simulink model "PEMFC_system"  (R2014b)
settings: Solver=ode45  StartTime=0.0  StopTime=10.0  RelTol=1e-3
settings Model: Creator=DELL  LastModifiedBy=dell

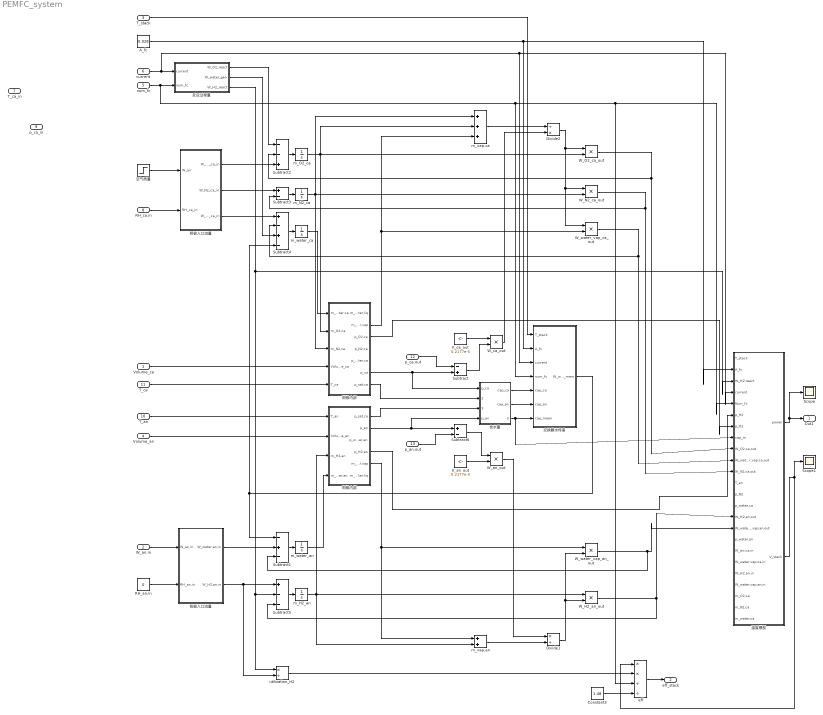
== system PEMFC_system ==
  Volume_ca : Inport
  W_an,in : Inport  Port=2
  T_stack : Inport  Port=3
  Volume_an : Inport  Port=4
  num_fc : Inport  Port=5
  current : Inport  Port=6
  T_ca_in : Inport  Port=7
  RH_ca,in : Inport  Port=8
  p_ca_in : Inport  Port=9
  T_an : Inport  Port=10
  T_ca : Inport  Port=11
  p_ca,out : Inport  Port=12
  p_an,out : Inport  Port=13
  A_fc : Constant  Value=0.028
  Constant3 : Constant  Value=1.48
  Divide1 : Product  Inputs=*/
  Divide2 : Product  Inputs=/*
  K_an_out : Constant  Value=0.2177e-5
  K_ca_out : Constant  Value=0.2177e-5
  RH_an,in : Constant  Value=0
  Scope : Scope
  Scope1 : Scope
  Subtract : Sum  Inputs=-+
  Subtract1 : Sum  Inputs=-+-
  Subtract2 : Sum  Inputs=--+
  Subtract3 : Sum  Inputs=+-
  Subtract4 : Sum  Inputs=+-+-
  Subtract5 : Sum  Inputs=+--
  Subtract6 : Sum  Inputs=+-
  W_H2_an_out : Product
  W_N2_ca_out : Product
  W_O2_ca_out : Product
  W_an_out : Product
  W_ca_out : Product
  W_water_vap_an_out : Product
  W_water_vap_ca_out : Product
  eff : Product  Inputs=**//
  m_H2_an : Integrator
  m_N2_ca : Integrator
  m_O2_ca : Integrator
  m_vap,an : Sum
  m_vap,ca : Sum  Inputs=+++
  m_water_an : Integrator
  m_water_ca : Integrator
  utilization_H2 : Product  Inputs=*/
  交换膜水传递 : Subsystem  TreatAsAtomicUnit=on
  反应过程量 : Subsystem
  含水量 : Subsystem
  温度模型 : Subsystem
  空气质量 : Step  SampleTime=0
  阳极入口流量 : Subsystem
  阳极内部 : Subsystem
  阴极入口流量 : Subsystem  TreatAsAtomicUnit=on
  阴极内部 : Subsystem
  Out1 : Outport
  eff_stack : Outport  Port=2
  wires:
  温度模型/1(power) -> Scope/1, Out1/1
  温度模型/2(V_stack) -> Scope1/1, eff/1
  current/1 -> 温度模型/4(current), 交换膜水传递/3(current), 反应过程量/1(current)
  Volume_ca/1 -> 阴极内部/4(Volume_ca)
  阴极内部/6(p_ca) -> 含水量/1(p_ca), Subtract/2
  Subtract/1 -> W_ca_out/2
  K_ca_out/1 -> W_ca_out/1
  阴极入口流量/1(W_O2_ca_in) -> Subtract2/3
  反应过程量/3(W_H2_react) -> utilization_H2/1, Subtract5/2, 温度模型/3(W_H2,react)
  反应过程量/1(W_O2_react) -> Subtract2/1
  Subtract2/1 -> m_O2_ca/1
  阴极入口流量/2(W_N2_ca_in) -> Subtract3/1
  Subtract3/1 -> m_N2_ca/1
  阴极入口流量/3(W_water_ca_in) -> Subtract4/1
  Subtract4/1 -> m_water_ca/1
  反应过程量/2(W_water_gen) -> Subtract4/3
  m_O2_ca/1 -> W_O2_ca_out/2, m_vap,ca/2, 阴极内部/2(m_O2,ca)
  m_N2_ca/1 -> W_N2_ca_out/2, m_vap,ca/1, 阴极内部/3(m_N2,ca)
  T_stack/1 -> 交换膜水传递/1(T_stack)
  阴极内部/2(m_water,vap) -> W_water_vap_ca_out/2, m_vap,ca/3
  m_water_ca/1 -> 阴极内部/1(m_water,ca)
  m_vap,ca/1 -> Divide2/1
  W_ca_out/1 -> Divide2/2
  Divide2/1 -> W_water_vap_ca_out/1, W_N2_ca_out/1, W_O2_ca_out/1
  W_O2_ca_out/1 -> 温度模型/9(W_O2,ca,out), Subtract2/2
  W_N2_ca_out/1 -> 温度模型/11(W_N2,ca,out), Subtract3/2
  W_water_vap_ca_out/1 -> Subtract4/2, 温度模型/10(W_water,vap,ca,out)
  交换膜水传递/1(W_water_mem) -> Subtract1/1, Subtract4/4
  W_an,in/1 -> 阳极入口流量/1(W_an,in)
  RH_an,in/1 -> 阳极入口流量/2(RH_an,in)
  阳极入口流量/2(W_H2,an,in) -> utilization_H2/2, Subtract5/1
  Subtract5/1 -> m_H2_an/1
  Subtract1/1 -> m_water_an/1
  阳极内部/4(p_H2,an) -> 温度模型/6(p_H2)
  Volume_an/1 -> 阳极内部/2(Volume_an)
  Subtract6/1 -> W_an_out/1
  K_an_out/1 -> W_an_out/2
  阳极内部/5(m_water,vap) -> W_water_vap_an_out/1, m_vap,an/1
  m_H2_an/1 -> W_H2_an_out/1, m_vap,an/2, 阳极内部/3(m_H2,an)
  W_an_out/1 -> Divide1/1
  m_vap,an/1 -> Divide1/2
  m_water_an/1 -> 阳极内部/4(m_water,an)
  Divide1/1 -> W_water_vap_an_out/2, W_H2_an_out/2
  阳极入口流量/1(W_water,an,in) -> Subtract1/2
  W_water_vap_an_out/1 -> 温度模型/16(W_water,vap,an,out), Subtract1/3
  W_H2_an_out/1 -> Subtract5/3, 温度模型/15(W_H2,an,out)
  阳极内部/2(p_an) -> Subtract6/1, 含水量/4(p_an)
  含水量/3(cap_mean) -> 交换膜水传递/7(cap_mean), 温度模型/8(cap_m)
  含水量/1(cap_ca) -> 交换膜水传递/5(cap_ca)
  含水量/2(cap_an) -> 交换膜水传递/6(cap_an)
  A_fc/1 -> 温度模型/2(A_fc), 交换膜水传递/2(A_fc)
  utilization_H2/1 -> eff/2
  num_fc/1 -> 反应过程量/2(num_fc), 交换膜水传递/4(num_fc), 温度模型/5(Num_fc), eff/3
  Constant3/1 -> eff/4
  eff/1 -> eff_stack/1
  空气质量/1 -> 阴极入口流量/1(W_air)
  阴极内部/3(p_O2,ca) -> 温度模型/7(p_O2)
  RH_ca,in/1 -> 阴极入口流量/2(RH_ca_in)
  T_an/1 -> 阳极内部/1(T_an)
  T_ca/1 -> 阴极内部/5(T_ca)
  阴极内部/7(p_sat,ca) -> 含水量/2(p_sat,ca)
  阳极内部/1(p_sat,ca) -> 含水量/3(p_sat,an)
  p_ca,out/1 -> Subtract/1
  p_an,out/1 -> Subtract6/2

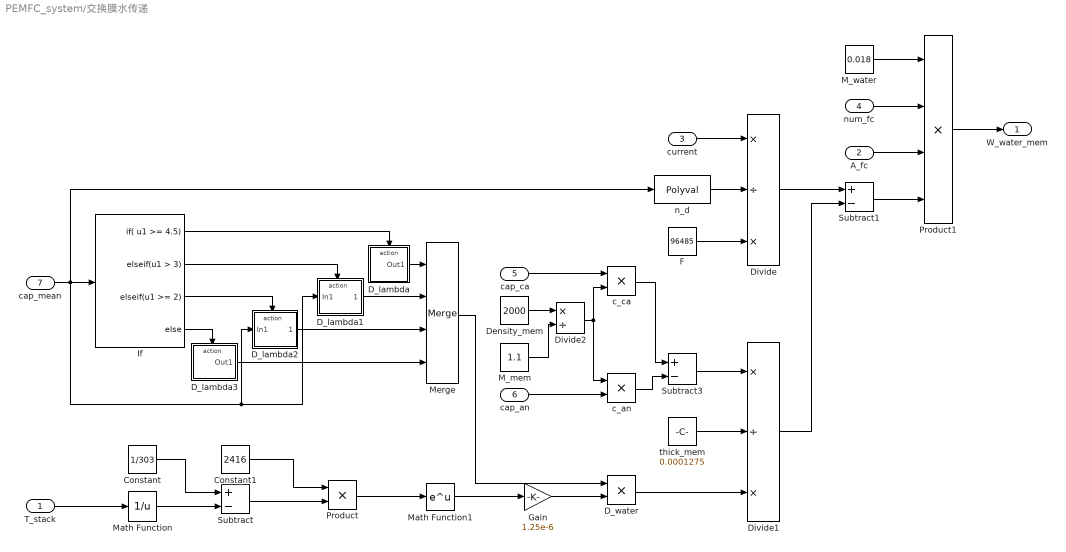
== system PEMFC_system/交换膜水传递 ==
  T_stack : Inport
  A_fc : Inport  Port=2
  current : Inport  Port=3
  num_fc : Inport  Port=4
  cap_ca : Inport  Port=5
  cap_an : Inport  Port=6
  cap_mean : Inport  Port=7
  Constant : Constant  Value=1/303
  Constant1 : Constant  Value=2416
  D_lambda : Subsystem  TreatAsAtomicUnit=on
  D_lambda1 : Subsystem  TreatAsAtomicUnit=on
  D_lambda2 : Subsystem  TreatAsAtomicUnit=on
  D_lambda3 : Subsystem  TreatAsAtomicUnit=on
  D_water : Product
  Density_mem : Constant  Value=2000
  Divide : Product  Inputs=*/*
  Divide1 : Product  Inputs=*/*
  Divide2 : Product  Inputs=*/
  F : Constant  Value=96485
  Gain : Gain  Gain=1.25e-6
  If : If  IfExpression=u1 >= 4.5  ElseIfExpressions=u1 > 3,u1 >= 2  ZeroCross=off
  M_mem : Constant  Value=1.1
  M_water : Constant  Value=0.018
  Math Function : Math  Operator=reciprocal  SaturateOnIntegerOverflow=on
  Math Function1 : Math  SaturateOnIntegerOverflow=on
  Merge : Merge  Inputs=4
  Product : Product
  Product1 : Product  Inputs=4
  Subtract : Sum  Inputs=+-
  Subtract1 : Sum  Inputs=+-
  Subtract3 : Sum  Inputs=+-
  c_an : Product
  c_ca : Product
  n_d : Polyval  Coefs=[0.0029,0.05,-3.4e-19]
  thick_mem : Constant  Value=0.0001275
  W_water_mem : Outport
  wires:
  If/1 -> D_lambda/Action
  If/2 -> D_lambda1/Action
  If/3 -> D_lambda2/Action
  If/4 -> D_lambda3/Action
  D_lambda/1(Out1) -> Merge/1
  D_lambda1/1(Out1) -> Merge/2
  D_lambda2/1(Out1) -> Merge/3
  D_lambda3/1(Out1) -> Merge/4
  T_stack/1 -> Math Function/1
  Math Function/1 -> Subtract/2
  Constant/1 -> Subtract/1
  Subtract/1 -> Product/2
  Constant1/1 -> Product/1
  Product/1 -> Math Function1/1
  Math Function1/1 -> Gain/1
  Merge/1 -> D_water/1
  cap_mean/1 -> n_d/1, D_lambda1/1(In1), D_lambda2/1(In1), If/1
  n_d/1 -> Divide/2
  F/1 -> Divide/3
  current/1 -> Divide/1
  cap_ca/1 -> c_ca/1
  Divide/1 -> Subtract1/1
  Divide1/1 -> Subtract1/2
  D_water/1 -> Divide1/3
  thick_mem/1 -> Divide1/2
  Subtract3/1 -> Divide1/1
  Subtract1/1 -> Product1/4
  A_fc/1 -> Product1/3
  num_fc/1 -> Product1/2
  M_water/1 -> Product1/1
  Product1/1 -> W_water_mem/1
  M_mem/1 -> Divide2/2
  Density_mem/1 -> Divide2/1
  Divide2/1 -> c_an/1, c_ca/2
  c_an/1 -> Subtract3/2
  c_ca/1 -> Subtract3/1
  cap_an/1 -> c_an/2
  Gain/1 -> D_water/2

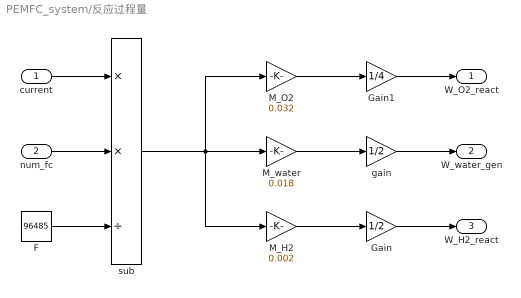
== system PEMFC_system/反应过程量 ==
  current : Inport
  num_fc : Inport  Port=2
  F : Constant  Value=96485
  Gain : Gain  Gain=1/2
  Gain1 : Gain  Gain=1/4
  M_H2 : Gain  Gain=0.002
  M_O2 : Gain  Gain=0.032
  M_water : Gain  Gain=0.018
  gain : Gain  Gain=1/2
  sub : Product  Inputs=**/
  W_O2_react : Outport
  W_water_gen : Outport  Port=2
  W_H2_react : Outport  Port=3
  wires:
  current/1 -> sub/1
  sub/1 -> M_water/1, M_O2/1, M_H2/1
  num_fc/1 -> sub/2
  F/1 -> sub/3
  M_H2/1 -> Gain/1
  Gain1/1 -> W_O2_react/1
  M_O2/1 -> Gain1/1
  Gain/1 -> W_H2_react/1
  M_water/1 -> gain/1
  gain/1 -> W_water_gen/1

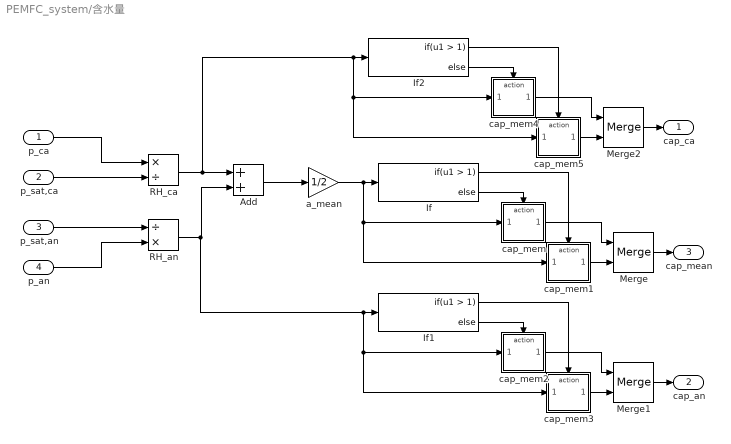
== system PEMFC_system/含水量 ==
  p_ca : Inport
  p_sat,ca : Inport  Port=2
  p_sat,an : Inport  Port=3
  p_an : Inport  Port=4
  Add : Sum
  If : If  IfExpression=u1 > 1
  If1 : If  IfExpression=u1 > 1
  If2 : If  IfExpression=u1 > 1
  Merge : Merge
  Merge1 : Merge
  Merge2 : Merge
  RH_an : Product  Inputs=/*
  RH_ca : Product  Inputs=*/
  a_mean : Gain  Gain=1/2
  cap_mem : Subsystem  TreatAsAtomicUnit=on
  cap_mem1 : Subsystem  TreatAsAtomicUnit=on
  cap_mem2 : Subsystem  TreatAsAtomicUnit=on
  cap_mem3 : Subsystem  TreatAsAtomicUnit=on
  cap_mem4 : Subsystem  TreatAsAtomicUnit=on
  cap_mem5 : Subsystem  TreatAsAtomicUnit=on
  cap_ca : Outport
  cap_an : Outport  Port=2
  cap_mean : Outport  Port=3
  wires:
  Add/1 -> a_mean/1
  cap_mem/1(Out1) -> Merge/1
  a_mean/1 -> cap_mem1/1(In1), cap_mem/1(In1), If/1
  Merge/1 -> cap_mean/1
  If/2 -> cap_mem/Action
  p_ca/1 -> RH_ca/1
  cap_mem1/1(Out1) -> Merge/2
  If/1 -> cap_mem1/Action
  p_sat,ca/1 -> RH_ca/2
  p_an/1 -> RH_an/2
  cap_mem2/1(Out1) -> Merge1/1
  RH_an/1 -> cap_mem3/1(In1), cap_mem2/1(In1), If1/1, Add/2
  Merge1/1 -> cap_an/1
  If1/2 -> cap_mem2/Action
  cap_mem3/1(Out1) -> Merge1/2
  If1/1 -> cap_mem3/Action
  cap_mem4/1(Out1) -> Merge2/1
  RH_ca/1 -> cap_mem5/1(In1), cap_mem4/1(In1), If2/1, Add/1
  Merge2/1 -> cap_ca/1
  If2/2 -> cap_mem4/Action
  cap_mem5/1(Out1) -> Merge2/2
  If2/1 -> cap_mem5/Action
  p_sat,an/1 -> RH_an/1

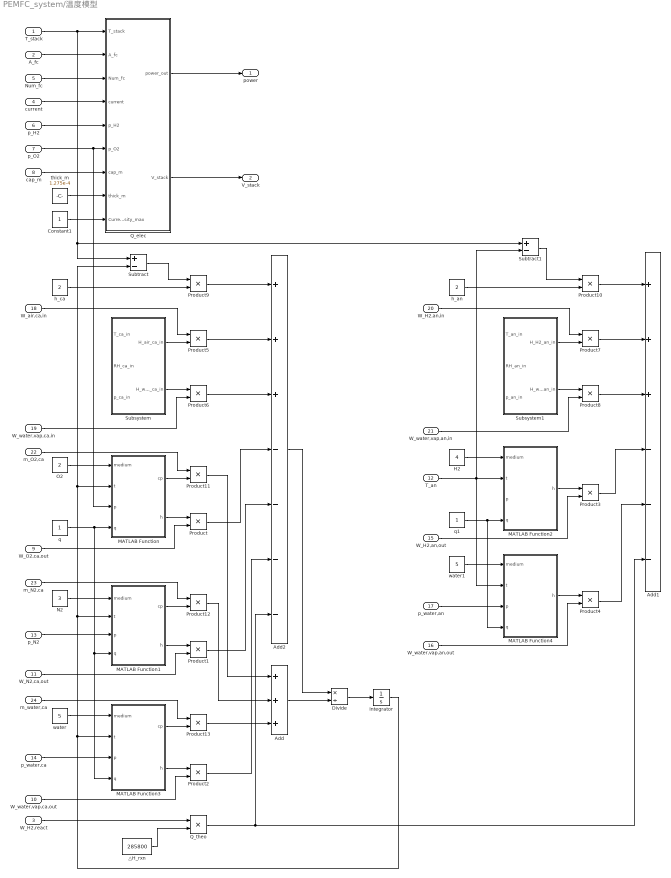
== system PEMFC_system/温度模型 ==
  T_stack : Inport
  A_fc : Inport  Port=2
  W_H2,react : Inport  Port=3
  current : Inport  Port=4
  Num_fc : Inport  Port=5
  p_H2 : Inport  Port=6
  p_O2 : Inport  Port=7
  cap_m : Inport  Port=8
  W_O2,ca,out : Inport  Port=9
  W_water,vap,ca,out : Inport  Port=10
  W_N2,ca,out : Inport  Port=11
  T_an : Inport  Port=12
  p_N2 : Inport  Port=13
  p_water,ca : Inport  Port=14
  W_H2,an,out : Inport  Port=15
  W_water,vap,an,out : Inport  Port=16
  p_water,an : Inport  Port=17
  W_air,ca,in : Inport  Port=18
  W_water,vap,ca,in : Inport  Port=19
  W_H2,an,in : Inport  Port=20
  W_water,vap,an,in : Inport  Port=21
  m_O2,ca : Inport  Port=22
  m_N2,ca : Inport  Port=23
  m_water,ca : Inport  Port=24
  Add : Sum  Inputs=3
  Add1 : Sum  Inputs=+++---
  Add2 : Sum  Inputs=+++----
  Constant1 : Constant
  Divide : Product  Inputs=*/
  H2 : Constant  Value=4
  Integrator : Integrator
  MATLAB Function : MATLAB Function  TreatAsAtomicUnit=on
  MATLAB Function1 : MATLAB Function  TreatAsAtomicUnit=on
  MATLAB Function2 : MATLAB Function  TreatAsAtomicUnit=on
  MATLAB Function3 : MATLAB Function  TreatAsAtomicUnit=on
  MATLAB Function4 : MATLAB Function  TreatAsAtomicUnit=on
  N2 : Constant  Value=3
  O2 : Constant  Value=2
  Product{,1..13} (14 alike) : Product
  Q_elec : Subsystem
  Q_theo : Product
  Subsystem : Subsystem
  Subsystem1 : Subsystem
  Subtract : Sum  Inputs=+-
  Subtract1 : Sum  Inputs=+-
  h_an : Constant  Value=2
  h_ca : Constant  Value=2
  q : Constant
  q1 : Constant
  thick_m : Constant  Value=1.275e-4
  water : Constant  Value=5
  water1 : Constant  Value=5
  △H_rxn : Constant  Value=285800
  power : Outport
  V_stack : Outport  Port=2
  wires:
  W_H2,react/1 -> Q_theo/1
  current/1 -> Q_elec/4(current)
  p_H2/1 -> Q_elec/5(p_H2)
  Q_elec/2(V_stack) -> V_stack/1
  △H_rxn/1 -> Q_theo/2
  Num_fc/1 -> Q_elec/3(Num_fc)
  cap_m/1 -> Q_elec/7(cap_m)
  thick_m/1 -> Q_elec/8(thick_m)
  A_fc/1 -> Q_elec/2(A_fc)
  Constant1/1 -> Q_elec/9(CurrentDensity_max)
  W_O2,ca,out/1 -> Product/2
  O2/1 -> MATLAB Function/1(medium)
  N2/1 -> MATLAB Function1/1(medium)
  H2/1 -> MATLAB Function2/1(medium)
  water/1 -> MATLAB Function3/1(medium)
  p_N2/1 -> MATLAB Function1/3(p)
  p_water,ca/1 -> MATLAB Function3/3(p)
  MATLAB Function/2(h) -> Product/1
  MATLAB Function1/2(h) -> Product1/1
  W_N2,ca,out/1 -> Product1/2
  MATLAB Function3/2(h) -> Product2/1
  W_water,vap,ca,out/1 -> Product2/2
  MATLAB Function2/1(h) -> Product3/1
  W_H2,an,out/1 -> Product3/2
  water1/1 -> MATLAB Function4/1(medium)
  p_water,an/1 -> MATLAB Function4/3(p)
  MATLAB Function4/1(h) -> Product4/1
  W_water,vap,an,out/1 -> Product4/2
  Subsystem/1(H_air_ca_in) -> Product5/2
  Subsystem/2(H_water_ca_in) -> Product6/1
  W_air,ca,in/1 -> Product5/1
  W_water,vap,ca,in/1 -> Product6/2
  Product5/1 -> Add2/2
  Product6/1 -> Add2/3
  Product/1 -> Add2/4
  Product1/1 -> Add2/5
  Product2/1 -> Add2/6
  Subsystem1/1(H_H2_an_in) -> Product7/2
  W_H2,an,in/1 -> Product7/1
  Subsystem1/2(H_water_an_in) -> Product8/1
  W_water,vap,an,in/1 -> Product8/2
  Integrator/1 -> Subtract/2, MATLAB Function/2(t), MATLAB Function1/2(t), MATLAB Function3/2(t)
  q/1 -> MATLAB Function3/4(q), MATLAB Function1/4(q), MATLAB Function/4(q)
  Product7/1 -> Add1/2
  Product8/1 -> Add1/3
  Product3/1 -> Add1/4
  Product4/1 -> Add1/5
  Q_theo/1 -> Add2/7, Add1/6
  T_stack/1 -> Subtract/1, Subtract1/1, Q_elec/1(T_stack)
  Subtract/1 -> Product9/1
  h_ca/1 -> Product9/2
  h_an/1 -> Product10/2
  Subtract1/1 -> Product10/1
  T_an/1 -> Subtract1/2, MATLAB Function2/2(t), MATLAB Function4/2(t)
  Product9/1 -> Add2/1
  Product10/1 -> Add1/1
  Q_elec/1(power_out) -> power/1
  p_O2/1 -> MATLAB Function/3(p), Q_elec/6(p_O2)
  q1/1 -> MATLAB Function4/4(q), MATLAB Function2/4(q)
  m_O2,ca/1 -> Product11/1
  MATLAB Function/1(cp) -> Product11/2
  m_N2,ca/1 -> Product12/1
  MATLAB Function1/1(cp) -> Product12/2
  m_water,ca/1 -> Product13/1
  MATLAB Function3/1(cp) -> Product13/2
  Product13/1 -> Add/3
  Product12/1 -> Add/2
  Product11/1 -> Add/1
  Add/1 -> Divide/2
  Add2/1 -> Divide/1
  Divide/1 -> Integrator/1

== system PEMFC_system/阳极入口流量 ==
  W_an,in : Inport
  RH_an,in : Inport  Port=2
  Constant1 : Constant
  W_H2_in : Product
  W_water_in : Product
  x_H2 : Sum  Inputs=+-
  W_water,an,in : Outport
  W_H2,an,in : Outport  Port=2
  wires:
  W_an,in/1 -> W_water_in/1, W_H2_in/1
  RH_an,in/1 -> W_water_in/2, x_H2/2
  Constant1/1 -> x_H2/1
  x_H2/1 -> W_H2_in/2
  W_H2_in/1 -> W_H2,an,in/1
  W_water_in/1 -> W_water,an,in/1

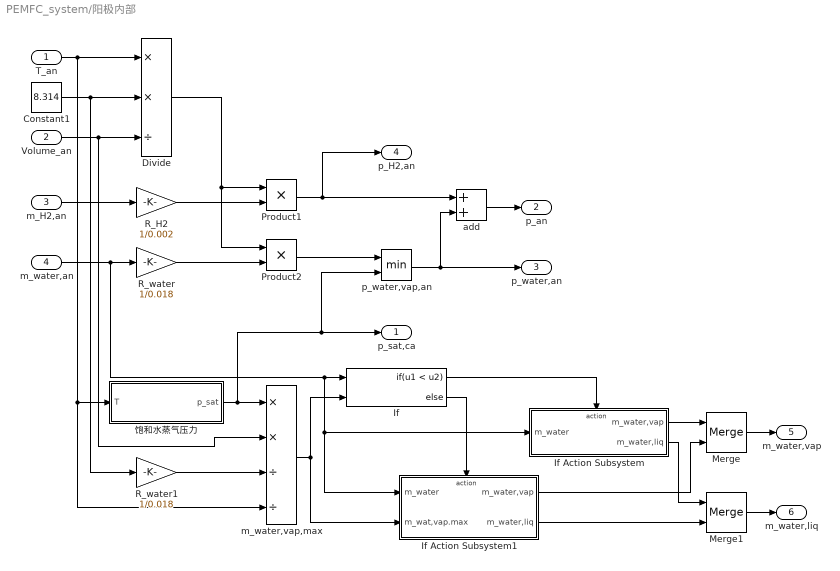
== system PEMFC_system/阳极内部 ==
  T_an : Inport
  Volume_an : Inport  Port=2
  m_H2,an : Inport  Port=3
  m_water,an : Inport  Port=4
  Constant1 : Constant  Value=8.314
  Divide : Product  Inputs=**/
  If : If  NumInputs=2  IfExpression=u1 < u2
  If Action Subsystem : Subsystem  TreatAsAtomicUnit=on
  If Action Subsystem1 : Subsystem  TreatAsAtomicUnit=on
  Merge : Merge
  Merge1 : Merge
  Product1 : Product
  Product2 : Product
  R_H2 : Gain  Gain=1/0.002
  R_water : Gain  Gain=1/0.018
  R_water1 : Gain  Gain=1/0.018
  add : Sum
  m_water,vap,max : Product  Inputs=**//
  p_water,vap,an : MinMax  Inputs=2
  饱和水蒸气压力 : Subsystem
  p_sat,ca : Outport
  p_an : Outport  Port=2
  p_water,an : Outport  Port=3
  p_H2,an : Outport  Port=4
  m_water,vap : Outport  Port=5
  m_water,liq : Outport  Port=6
  wires:
  Constant1/1 -> R_water1/1, Divide/2
  m_H2,an/1 -> R_H2/1
  R_H2/1 -> Product1/2
  R_water/1 -> Product2/2
  Product1/1 -> add/1, p_H2,an/1
  Product2/1 -> p_water,vap,an/1
  Divide/1 -> Product2/1, Product1/1
  饱和水蒸气压力/1(p_sat) -> p_water,vap,an/2, p_sat,ca/1, m_water,vap,max/1
  Volume_an/1 -> m_water,vap,max/2, Divide/3
  R_water1/1 -> m_water,vap,max/3
  T_an/1 -> m_water,vap,max/4, 饱和水蒸气压力/1(T), Divide/1
  m_water,an/1 -> If Action Subsystem1/1(m_water), If Action Subsystem/1(m_water), If/1, R_water/1
  m_water,vap,max/1 -> If/2, If Action Subsystem1/2(m_wat,vap.max)
  If/1 -> If Action Subsystem/Action
  If/2 -> If Action Subsystem1/Action
  If Action Subsystem/1(m_water,vap) -> Merge/1
  If Action Subsystem1/1(m_water,vap) -> Merge/2
  If Action Subsystem1/2(m_water,liq) -> Merge1/2
  If Action Subsystem/2(m_water,liq) -> Merge1/1
  Merge/1 -> m_water,vap/1
  Merge1/1 -> m_water,liq/1
  p_water,vap,an/1 -> p_water,an/1, add/2
  add/1 -> p_an/1

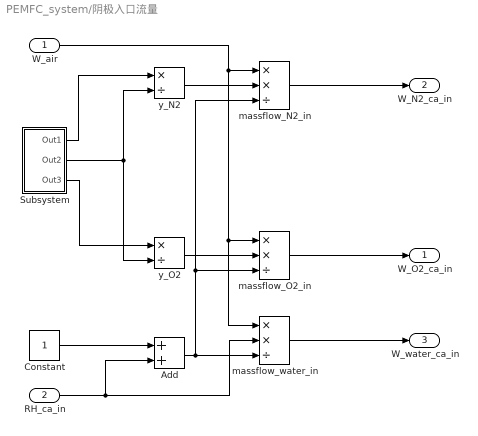
== system PEMFC_system/阴极入口流量 ==
  W_air : Inport
  RH_ca_in : Inport  Port=2
  Add : Sum
  Constant : Constant
  Subsystem : Subsystem
  massflow_N2_in : Product  Inputs=**/
  massflow_O2_in : Product  Inputs=**/
  massflow_water_in : Product  Inputs=**/
  y_N2 : Product  Inputs=*/
  y_O2 : Product  Inputs=*/
  W_O2_ca_in : Outport
  W_N2_ca_in : Outport  Port=2
  W_water_ca_in : Outport  Port=3
  wires:
  RH_ca_in/1 -> Add/2, massflow_water_in/2
  W_air/1 -> massflow_water_in/1, massflow_O2_in/1, massflow_N2_in/1
  y_N2/1 -> massflow_N2_in/2
  Add/1 -> massflow_water_in/3, massflow_N2_in/3, massflow_O2_in/3
  y_O2/1 -> massflow_O2_in/2
  massflow_N2_in/1 -> W_N2_ca_in/1
  massflow_O2_in/1 -> W_O2_ca_in/1
  massflow_water_in/1 -> W_water_ca_in/1
  Subsystem/2(Out2) -> y_O2/2, y_N2/2
  Subsystem/1(Out1) -> y_N2/1
  Subsystem/3(Out3) -> y_O2/1
  Constant/1 -> Add/1

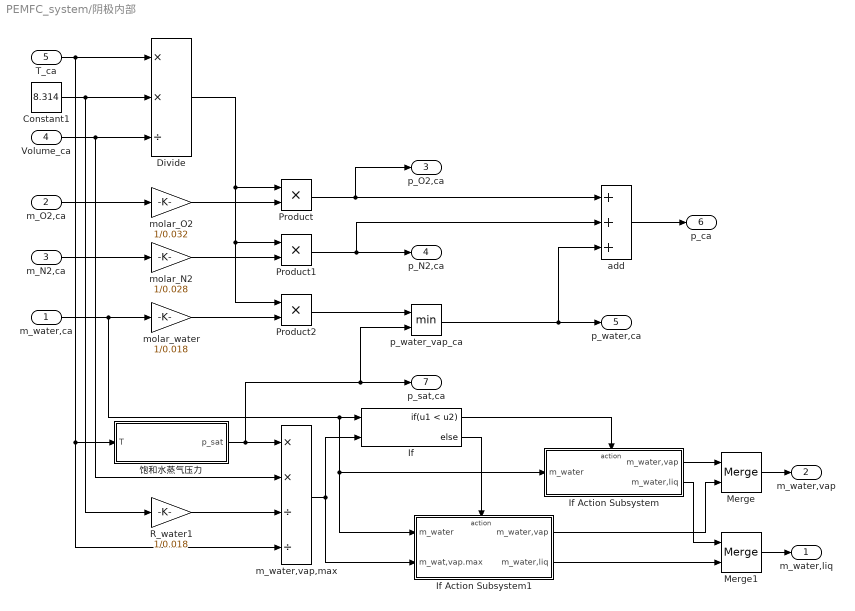
== system PEMFC_system/阴极内部 ==
  m_water,ca : Inport
  m_O2,ca : Inport  Port=2
  m_N2,ca : Inport  Port=3
  Volume_ca : Inport  Port=4
  T_ca : Inport  Port=5
  Constant1 : Constant  Value=8.314
  Divide : Product  Inputs=**/
  If : If  NumInputs=2  IfExpression=u1 < u2
  If Action Subsystem : Subsystem  TreatAsAtomicUnit=on
  If Action Subsystem1 : Subsystem  TreatAsAtomicUnit=on
  Merge : Merge
  Merge1 : Merge
  Product : Product
  Product1 : Product
  Product2 : Product
  R_water1 : Gain  Gain=1/0.018
  add : Sum  Inputs=3
  m_water,vap,max : Product  Inputs=**//
  molar_N2 : Gain  Gain=1/0.028
  molar_O2 : Gain  Gain=1/0.032
  molar_water : Gain  Gain=1/0.018
  p_water_vap_ca : MinMax  Inputs=2
  饱和水蒸气压力 : Subsystem
  m_water,liq : Outport
  m_water,vap : Outport  Port=2
  p_O2,ca : Outport  Port=3
  p_N2,ca : Outport  Port=4
  p_water,ca : Outport  Port=5
  p_ca : Outport  Port=6
  p_sat,ca : Outport  Port=7
  wires:
  m_O2,ca/1 -> molar_O2/1
  m_N2,ca/1 -> molar_N2/1
  molar_O2/1 -> Product/2
  Divide/1 -> Product/1, Product1/1, Product2/1
  Product/1 -> add/1, p_O2,ca/1
  molar_N2/1 -> Product1/2
  molar_water/1 -> Product2/2
  Product1/1 -> add/2, p_N2,ca/1
  Constant1/1 -> Divide/2, R_water1/1
  饱和水蒸气压力/1(p_sat) -> p_sat,ca/1, p_water_vap_ca/2, m_water,vap,max/1
  Volume_ca/1 -> Divide/3, m_water,vap,max/2
  R_water1/1 -> m_water,vap,max/3
  T_ca/1 -> Divide/1, 饱和水蒸气压力/1(T), m_water,vap,max/4
  m_water,ca/1 -> molar_water/1, If Action Subsystem1/1(m_water), If Action Subsystem/1(m_water), If/1
  m_water,vap,max/1 -> If/2, If Action Subsystem1/2(m_wat,vap.max)
  If/1 -> If Action Subsystem/Action
  If/2 -> If Action Subsystem1/Action
  If Action Subsystem/1(m_water,vap) -> Merge/1
  If Action Subsystem1/1(m_water,vap) -> Merge/2
  If Action Subsystem1/2(m_water,liq) -> Merge1/2
  If Action Subsystem/2(m_water,liq) -> Merge1/1
  Merge/1 -> m_water,vap/1
  Merge1/1 -> m_water,liq/1
  Product2/1 -> p_water_vap_ca/1
  p_water_vap_ca/1 -> p_water,ca/1, add/3
  add/1 -> p_ca/1

== system PEMFC_system/交换膜水传递/D_lambda ==
  Action Port : ActionPort  ActionType=then
  Constant : Constant  Value=1.25e-6
  Out1 : Outport
  wires:
  Constant/1 -> Out1/1

== system PEMFC_system/交换膜水传递/D_lambda1 ==
  In1 : Inport
  Action Port : ActionPort  ActionType=elseif
  Constant : Constant  Value=3
  Constant1 : Constant  Value=1.67
  Gain : Gain  Gain=1e-6
  Product : Product
  Subtract : Sum  Inputs=+-
  Subtract1 : Sum  Inputs=+-
  Out1 : Outport
  wires:
  In1/1 -> Subtract/1
  Constant/1 -> Subtract/2, Subtract1/1
  Constant1/1 -> Product/1
  Subtract/1 -> Product/2
  Product/1 -> Subtract1/2
  Subtract1/1 -> Gain/1
  Gain/1 -> Out1/1

== system PEMFC_system/交换膜水传递/D_lambda2 ==
  In1 : Inport
  Action Port : ActionPort  ActionType=elseif
  Add : Sum
  Constant : Constant  Value=2
  Constant1 : Constant
  Gain : Gain  Gain=1e-6
  Product : Product
  Subtract : Sum  Inputs=+-
  Out1 : Outport
  wires:
  In1/1 -> Subtract/1
  Constant/1 -> Product/2, Subtract/2
  Subtract/1 -> Product/1
  Product/1 -> Add/2
  Add/1 -> Gain/1
  Gain/1 -> Out1/1
  Constant1/1 -> Add/1

== system PEMFC_system/交换膜水传递/D_lambda3 ==
  Action Port : ActionPort  ActionType=else
  Constant : Constant  Value=1e-6
  Out1 : Outport
  wires:
  Constant/1 -> Out1/1

== system PEMFC_system/含水量/cap_mem ==
  In1 : Inport
  Action Port : ActionPort  ActionType=else
  Polynomial : Polyval  Coefs=[36,-39.85,17.81,0.043]
  Out1 : Outport
  wires:
  In1/1 -> Polynomial/1
  Polynomial/1 -> Out1/1

== system PEMFC_system/含水量/cap_mem1 ==
  In1 : Inport
  Action Port : ActionPort  ActionType=then
  Polynomial : Polyval  Coefs=[1.4,-14]
  Out1 : Outport
  wires:
  In1/1 -> Polynomial/1
  Polynomial/1 -> Out1/1

== system PEMFC_system/含水量/cap_mem2 ==
  In1 : Inport
  Action Port : ActionPort  ActionType=else
  Polynomial : Polyval  Coefs=[36,-39.85,17.81,0.043]
  Out1 : Outport
  wires:
  In1/1 -> Polynomial/1
  Polynomial/1 -> Out1/1

== system PEMFC_system/含水量/cap_mem3 ==
  In1 : Inport
  Action Port : ActionPort  ActionType=then
  Polynomial : Polyval  Coefs=[1.4,-14]
  Out1 : Outport
  wires:
  In1/1 -> Polynomial/1
  Polynomial/1 -> Out1/1

== system PEMFC_system/含水量/cap_mem4 ==
  In1 : Inport
  Action Port : ActionPort  ActionType=else
  Polynomial : Polyval  Coefs=[36,-39.85,17.81,0.043]
  Out1 : Outport
  wires:
  In1/1 -> Polynomial/1
  Polynomial/1 -> Out1/1

== system PEMFC_system/含水量/cap_mem5 ==
  In1 : Inport
  Action Port : ActionPort  ActionType=then
  Polynomial : Polyval  Coefs=[1.4,-14]
  Out1 : Outport
  wires:
  In1/1 -> Polynomial/1
  Polynomial/1 -> Out1/1

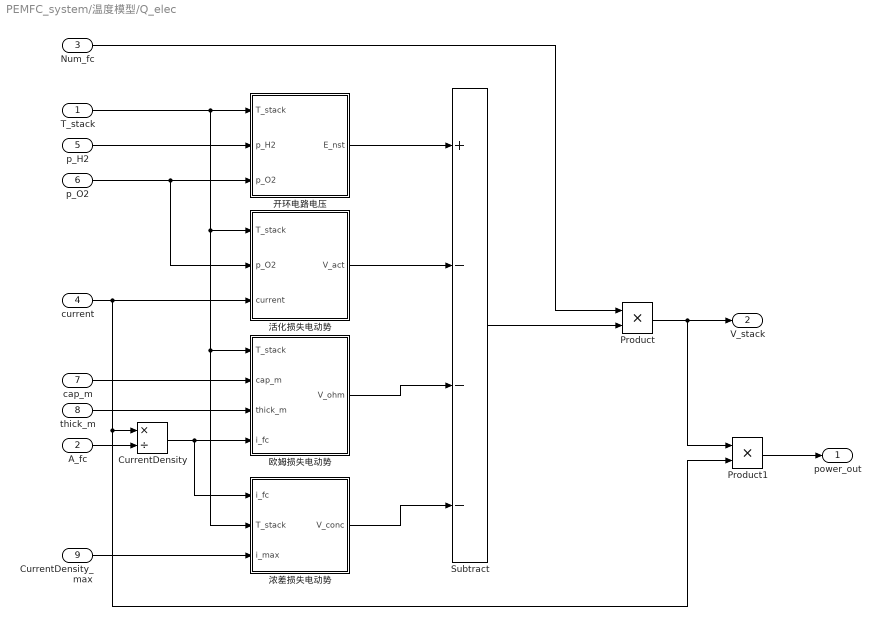
== system PEMFC_system/温度模型/Q_elec ==
  T_stack : Inport
  A_fc : Inport  Port=2
  Num_fc : Inport  Port=3
  current : Inport  Port=4
  p_H2 : Inport  Port=5
  p_O2 : Inport  Port=6
  cap_m : Inport  Port=7
  thick_m : Inport  Port=8
  CurrentDensity_max : Inport  Port=9
  CurrentDensity : Product  Inputs=*/
  Product : Product
  Product1 : Product
  Subtract : Sum  Inputs=+---
  开环电路电压 : Subsystem  TreatAsAtomicUnit=on
  欧姆损失电动势 : MATLAB Function  TreatAsAtomicUnit=on
  活化损失电动势 : MATLAB Function  TreatAsAtomicUnit=on
  浓差损失电动势 : Subsystem
  power_out : Outport
  V_stack : Outport  Port=2
  wires:
  p_H2/1 -> 开环电路电压/2(p_H2)
  p_O2/1 -> 活化损失电动势/2(p_O2), 开环电路电压/3(p_O2)
  T_stack/1 -> 开环电路电压/1(T_stack), 浓差损失电动势/2(T_stack), 欧姆损失电动势/1(T_stack), 活化损失电动势/1(T_stack)
  current/1 -> Product1/2, CurrentDensity/1, 活化损失电动势/3(current)
  cap_m/1 -> 欧姆损失电动势/2(cap_m)
  开环电路电压/1(E_nst) -> Subtract/1
  活化损失电动势/1(V_act) -> Subtract/2
  欧姆损失电动势/1(V_ohm) -> Subtract/3
  浓差损失电动势/1(V_conc) -> Subtract/4
  Subtract/1 -> Product/2
  Product/1 -> Product1/1, V_stack/1
  Product1/1 -> power_out/1
  Num_fc/1 -> Product/1
  thick_m/1 -> 欧姆损失电动势/3(thick_m)
  A_fc/1 -> CurrentDensity/2
  CurrentDensity/1 -> 浓差损失电动势/1(i_fc), 欧姆损失电动势/4(i_fc)
  CurrentDensity_max/1 -> 浓差损失电动势/3(i_max)

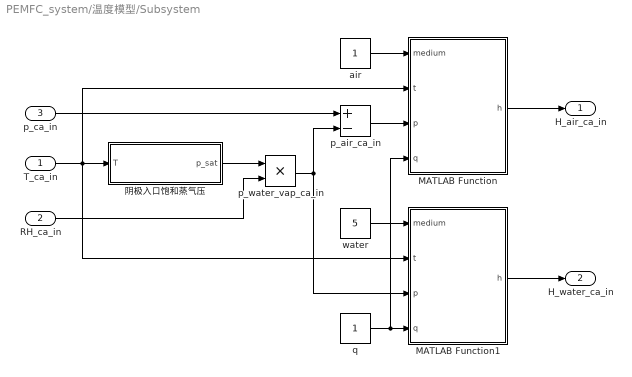
== system PEMFC_system/温度模型/Subsystem ==
  T_ca_in : Inport
  RH_ca_in : Inport  Port=2
  p_ca_in : Inport  Port=3
  MATLAB Function : MATLAB Function  TreatAsAtomicUnit=on
  MATLAB Function1 : MATLAB Function  TreatAsAtomicUnit=on
  air : Constant
  p_air_ca_in : Sum  Inputs=+-
  p_water_vap_ca_in : Product
  q : Constant
  water : Constant  Value=5
  阴极入口饱和蒸气压 : Subsystem
  H_air_ca_in : Outport
  H_water_ca_in : Outport  Port=2
  wires:
  阴极入口饱和蒸气压/1(p_sat) -> p_water_vap_ca_in/1
  RH_ca_in/1 -> p_water_vap_ca_in/2
  p_water_vap_ca_in/1 -> MATLAB Function1/3(p), p_air_ca_in/2
  MATLAB Function1/1(h) -> H_water_ca_in/1
  water/1 -> MATLAB Function1/1(medium)
  p_ca_in/1 -> p_air_ca_in/1
  p_air_ca_in/1 -> MATLAB Function/3(p)
  q/1 -> MATLAB Function/4(q), MATLAB Function1/4(q)
  MATLAB Function/1(h) -> H_air_ca_in/1
  air/1 -> MATLAB Function/1(medium)
  T_ca_in/1 -> MATLAB Function1/2(t), MATLAB Function/2(t), 阴极入口饱和蒸气压/1(T)

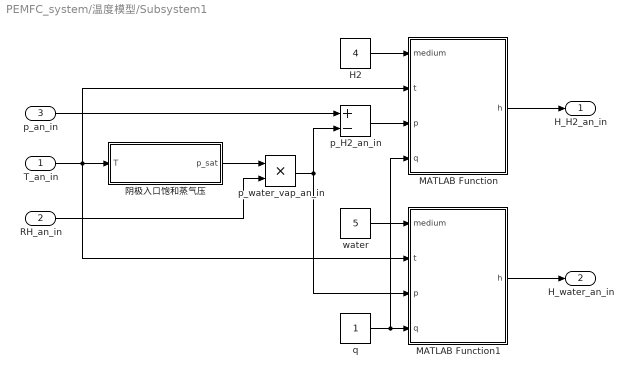
== system PEMFC_system/温度模型/Subsystem1 ==
  T_an_in : Inport
  RH_an_in : Inport  Port=2
  p_an_in : Inport  Port=3
  H2 : Constant  Value=4
  MATLAB Function : MATLAB Function  TreatAsAtomicUnit=on
  MATLAB Function1 : MATLAB Function  TreatAsAtomicUnit=on
  p_H2_an_in : Sum  Inputs=+-
  p_water_vap_an_in : Product
  q : Constant
  water : Constant  Value=5
  阴极入口饱和蒸气压 : Subsystem
  H_H2_an_in : Outport
  H_water_an_in : Outport  Port=2
  wires:
  阴极入口饱和蒸气压/1(p_sat) -> p_water_vap_an_in/1
  RH_an_in/1 -> p_water_vap_an_in/2
  p_water_vap_an_in/1 -> MATLAB Function1/3(p), p_H2_an_in/2
  MATLAB Function1/1(h) -> H_water_an_in/1
  water/1 -> MATLAB Function1/1(medium)
  p_an_in/1 -> p_H2_an_in/1
  p_H2_an_in/1 -> MATLAB Function/3(p)
  q/1 -> MATLAB Function/4(q), MATLAB Function1/4(q)
  MATLAB Function/1(h) -> H_H2_an_in/1
  H2/1 -> MATLAB Function/1(medium)
  T_an_in/1 -> MATLAB Function1/2(t), MATLAB Function/2(t), 阴极入口饱和蒸气压/1(T)

== system PEMFC_system/阳极内部/If Action Subsystem ==
  m_water : Inport
  Action Port : ActionPort
  Constant : Constant  Value=0
  m_water,vap : Outport
  m_water,liq : Outport  Port=2
  wires:
  m_water/1 -> m_water,vap/1
  Constant/1 -> m_water,liq/1

== system PEMFC_system/阳极内部/If Action Subsystem1 ==
  m_water : Inport
  m_wat,vap.max : Inport  Port=2
  Action Port : ActionPort
  Subtract : Sum  Inputs=+-
  m_water,vap : Outport
  m_water,liq : Outport  Port=2
  wires:
  m_water/1 -> Subtract/1
  m_wat,vap.max/1 -> m_water,vap/1, Subtract/2
  Subtract/1 -> m_water,liq/1

== system PEMFC_system/阳极内部/饱和水蒸气压力 ==
  T : Inport
  Constant : Constant  Value=273.15
  Math Function : Math  Operator=10^u  SaturateOnIntegerOverflow=on
  Polynomial : Polyval  Coefs=[1.4454e-7,-9.1837e-5,0.2953,-2.1794]
  substract : Sum  Inputs=+-
  p_sat : Outport
  wires:
  Polynomial/1 -> Math Function/1
  T/1 -> substract/1
  Math Function/1 -> p_sat/1
  substract/1 -> Polynomial/1
  Constant/1 -> substract/2

== system PEMFC_system/阴极入口流量/Subsystem ==
  M_N2 : Constant  Value=0.028
  M_O2 : Constant  Value=0.032
  M_air : Sum
  Product : Product
  Product1 : Product
  constant : Constant
  x_N2 : Sum  Inputs=+-
  x_O2 : Constant  Value=0.21
  Out1 : Outport
  Out2 : Outport  Port=2
  Out3 : Outport  Port=3
  wires:
  constant/1 -> x_N2/1
  x_O2/1 -> Product/1, x_N2/2
  M_O2/1 -> Product/2
  M_N2/1 -> Product1/1
  x_N2/1 -> Product1/2
  Product/1 -> Out3/1, M_air/2
  Product1/1 -> Out1/1, M_air/1
  M_air/1 -> Out2/1

== system PEMFC_system/阴极内部/If Action Subsystem ==
  m_water : Inport
  Action Port : ActionPort
  Constant : Constant  Value=0
  m_water,vap : Outport
  m_water,liq : Outport  Port=2
  wires:
  m_water/1 -> m_water,vap/1
  Constant/1 -> m_water,liq/1

== system PEMFC_system/阴极内部/If Action Subsystem1 ==
  m_water : Inport
  m_wat,vap.max : Inport  Port=2
  Action Port : ActionPort
  Subtract : Sum  Inputs=+-
  m_water,vap : Outport
  m_water,liq : Outport  Port=2
  wires:
  m_water/1 -> Subtract/1
  m_wat,vap.max/1 -> m_water,vap/1, Subtract/2
  Subtract/1 -> m_water,liq/1

== system PEMFC_system/阴极内部/饱和水蒸气压力 ==
  T : Inport
  Constant : Constant  Value=273.15
  Math Function : Math  Operator=10^u  SaturateOnIntegerOverflow=on
  Polynomial : Polyval  Coefs=[1.4454e-7,-9.1837e-5,0.2953,-2.1794]
  substract : Sum  Inputs=+-
  p_sat : Outport
  wires:
  Polynomial/1 -> Math Function/1
  T/1 -> substract/1
  Math Function/1 -> p_sat/1
  substract/1 -> Polynomial/1
  Constant/1 -> substract/2

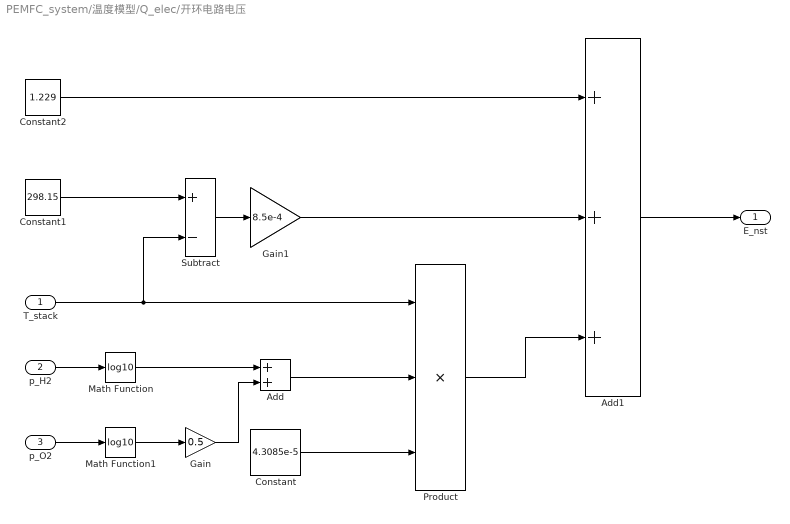
== system PEMFC_system/温度模型/Q_elec/开环电路电压 ==
  T_stack : Inport
  p_H2 : Inport  Port=2
  p_O2 : Inport  Port=3
  Add : Sum
  Add1 : Sum  Inputs=+++
  Constant : Constant  Value=4.3085e-5
  Constant1 : Constant  Value=298.15
  Constant2 : Constant  Value=1.229
  Gain : Gain  Gain=0.5
  Gain1 : Gain  Gain=8.5e-4
  Math Function : Math  Operator=log10  SaturateOnIntegerOverflow=on
  Math Function1 : Math  Operator=log10  SaturateOnIntegerOverflow=on
  Product : Product  Inputs=3
  Subtract : Sum  Inputs=+-
  E_nst : Outport
  wires:
  p_H2/1 -> Math Function/1
  p_O2/1 -> Math Function1/1
  Math Function1/1 -> Gain/1
  Gain/1 -> Add/2
  Math Function/1 -> Add/1
  T_stack/1 -> Subtract/2, Product/1
  Add/1 -> Product/2
  Constant/1 -> Product/3
  Constant1/1 -> Subtract/1
  Subtract/1 -> Gain1/1
  Constant2/1 -> Add1/1
  Gain1/1 -> Add1/2
  Product/1 -> Add1/3
  Add1/1 -> E_nst/1

== system PEMFC_system/温度模型/Q_elec/浓差损失电动势 ==
  i_fc : Inport
  T_stack : Inport  Port=2
  i_max : Inport  Port=3
  Divide : Product  Inputs=*/
  Divide1 : Product  Inputs=***//
  F : Constant  Value=96485
  Math Function : Math  Operator=log10  SaturateOnIntegerOverflow=on
  R : Constant  Value=8.314
  Subtract : Sum  Inputs=+-
  constant : Constant
  constant2 : Constant  Value=2
  V_conc : Outport
  wires:
  i_fc/1 -> Divide/1
  i_max/1 -> Divide/2
  constant/1 -> Subtract/1
  Divide/1 -> Subtract/2
  Divide1/1 -> V_conc/1
  Subtract/1 -> Math Function/1
  Math Function/1 -> Divide1/3
  R/1 -> Divide1/2
  T_stack/1 -> Divide1/1
  F/1 -> Divide1/4
  constant2/1 -> Divide1/5

== system PEMFC_system/温度模型/Subsystem/阴极入口饱和蒸气压 ==
  T : Inport
  Constant : Constant  Value=273.15
  Math Function : Math  Operator=10^u  SaturateOnIntegerOverflow=on
  Polynomial : Polyval  Coefs=[1.4454e-7,-9.1837e-5,0.2953,-2.1794]
  substract : Sum  Inputs=+-
  p_sat : Outport
  wires:
  Polynomial/1 -> Math Function/1
  T/1 -> substract/1
  Math Function/1 -> p_sat/1
  substract/1 -> Polynomial/1
  Constant/1 -> substract/2

== system PEMFC_system/温度模型/Subsystem1/阴极入口饱和蒸气压 ==
  T : Inport
  Constant : Constant  Value=273.15
  Math Function : Math  Operator=10^u  SaturateOnIntegerOverflow=on
  Polynomial : Polyval  Coefs=[1.4454e-7,-9.1837e-5,0.2953,-2.1794]
  substract : Sum  Inputs=+-
  p_sat : Outport
  wires:
  Polynomial/1 -> Math Function/1
  T/1 -> substract/1
  Math Function/1 -> p_sat/1
  substract/1 -> Polynomial/1
  Constant/1 -> substract/2

== matlab function PEMFC_system/温度模型/Q_elec/欧姆损失电动势 ==
  data: T_stack input; V_ohm output; cap_m input; thick_m input; i_fc input
function V_ohm = fcn( T_stack,cap_m,thick_m,i_fc )
b1=0.005139*cap_m-0.00326;
b2=1286;
cond_m=b1*exp(b2*(1/303-1/T_stack));
R_ohm=thick_m/cond_m;
V_ohm=i_fc*R_ohm;

== matlab function PEMFC_system/温度模型/Q_elec/活化损失电动势 ==
  data: T_stack input; V_act output; p_O2 input; current input
function V_act = fcn( T_stack,p_O2,current )
%#codegen
V_act=0.9514-3.12e-3*T_stack+1.87e-4*T_stack*ln(current)-7.4e-5*T_stack*ln(p_O2/(5.08e6*exp(-498/T_stack)));

== matlab function PEMFC_system/温度模型/MATLAB Function ==
  data: cp output; medium input; t input; p input; q input; h output
function [cp,h] = fcn(medium,t,p,q)
%#codegen
rho=1;
cv=1;
cp=1;
h=1;
k=1;
mu=1;
coder.extrinsic('props');
[ rho,cv,cp,h,mu,k ] = props( medium,t,p,q );

== matlab function PEMFC_system/温度模型/MATLAB Function1 ==
  data: cp output; medium input; t input; p input; q input; h output
function [cp,h] = fcn(medium,t,p,q)
%#codegen
rho=1;
cv=1;
cp=1;
h=1;
k=1;
mu=1;
coder.extrinsic('props');
[ rho,cv,cp,h,mu,k ] = props( medium,t,p,q );

== matlab function PEMFC_system/温度模型/MATLAB Function2 ==
  data: medium input; t input; p input; q input; h output
function h = fcn(medium,t,p,q)
%#codegen
rho=1;
cv=1;
cp=1;
h=1;
k=1;
mu=1;
coder.extrinsic('props');
[ rho,cv,cp,h,mu,k ] = props( medium,t,p,q );

== matlab function PEMFC_system/温度模型/MATLAB Function3 ==
  data: cp output; medium input; t input; p input; q input; h output
function [cp,h] = fcn(medium,t,p,q)
%#codegen
rho=1;
cv=1;
cp=1;
h=1;
k=1;
mu=1;
coder.extrinsic('props');
[ rho,cv,cp,h,mu,k ] = props( medium,t,p,q );

== matlab function PEMFC_system/温度模型/Subsystem1/MATLAB Function ==
  data: medium input; t input; p input; q input; h output
function h = fcn(medium,t,p,q)
%#codegen
rho=1;
cv=1;
cp=1;
h=1;
k=1;
mu=1;
coder.extrinsic('props');
[ rho,cv,cp,h,mu,k ] = props( medium,t,p,q );

== matlab function PEMFC_system/温度模型/Subsystem1/MATLAB Function1 ==
  data: medium input; t input; p input; q input; h output
function h = fcn(medium,t,p,q)
%#codegen
rho=1;
cv=1;
cp=1;
h=1;
k=1;
mu=1;
coder.extrinsic('props');
[ rho,cv,cp,h,mu,k ] = props( medium,t,p,q );

== matlab function PEMFC_system/温度模型/MATLAB Function4 ==
  data: medium input; t input; p input; q input; h output
function h = fcn(medium,t,p,q)
%#codegen
rho=1;
cv=1;
cp=1;
h=1;
k=1;
mu=1;
coder.extrinsic('props');
[ rho,cv,cp,h,mu,k ] = props( medium,t,p,q );

== matlab function PEMFC_system/温度模型/Subsystem/MATLAB Function ==
  data: medium input; t input; p input; q input; h output
function h = fcn(medium,t,p,q)
%#codegen
rho=1;
cv=1;
cp=1;
h=1;
k=1;
mu=1;
coder.extrinsic('props');
[ rho,cv,cp,h,mu,k ] = props( medium,t,p,q );

== matlab function PEMFC_system/温度模型/Subsystem/MATLAB Function1 ==
  data: medium input; t input; p input; q input; h output
function h = fcn(medium,t,p,q)
%#codegen
rho=1;
cv=1;
cp=1;
h=1;
k=1;
mu=1;
coder.extrinsic('props');
[ rho,cv,cp,h,mu,k ] = props( medium,t,p,q );
